simulink model "test"  (R2018b)
settings: Solver=FixedStepAuto  StartTime=1  StopTime=intervals  FixedStep=1  RelTol=1e-3
values from neighbouring files (symbols this model uses):
  intervals = days*288    (= 288)    [init.m]
settings Model: EnablePacing=on  PacingRate=30  Creator=rexlu  LastModifiedBy=hans

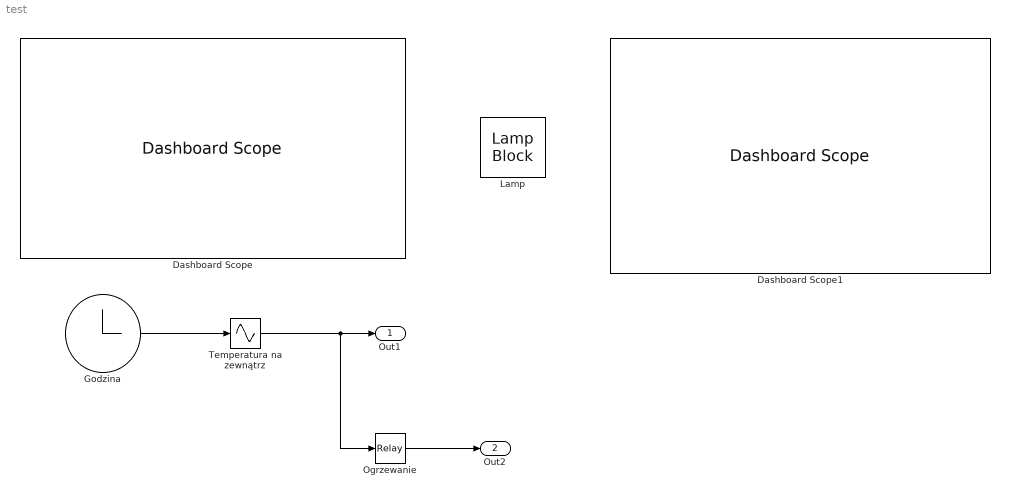
== system test ==
  Dashboard Scope : DashboardScope  WebBlockId=31  TimeSpan=288  Ymin=-15  Ymax=50  ScaleAtStop=off
  Dashboard Scope1 : DashboardScope  WebBlockId=45  TimeSpan=288  Ymin=0  Ymax=2
  "Godzina " : Clock
  Lamp : LampBlock  WebBlockId=33
  Ogrzewanie : Relay  OnSwitchValue=22  OffSwitchValue=18  OnOutputValue=0  OffOutputValue=1
  Temperatura na zewnątrz : Sin  TimeSource=Use external signal  Amplitude=18  Bias=10  Frequency=2*pi/intervals  Phase=-pi/2  SampleTime=0
  Out1 : Outport
  Out2 : Outport  Port=2
  wires:
  "Godzina "/1 -> Temperatura na zewnątrz/1
  Temperatura na zewnątrz/1 -> Ogrzewanie/1, Out1/1
  Ogrzewanie/1 -> Out2/1
